simulink model "Flyback_converter"  (R2022b)
settings: Solver=ode23t  StartTime=0.0  StopTime=.2  RelTol=1e-3
libraries: spsSeriesRLCBranchLib x5, spsCurrentMeasurementLib x2, spsVoltageMeasurementLib x2, spsDCVoltageSourceLib x1, spsDiodeLib x1, spsLinearTransformerLib x1, dspstat3 x1, spsMosfetLib x1, simulink x1, spspowerguiLib x1
settings Model: Creator=es-ahmedabdellatif20  LastModifiedBy=es-ahmedabdellatif20

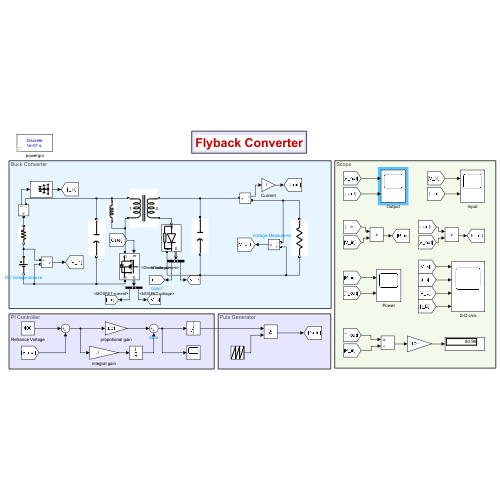
[thumbnail: Simulink's stored preview of the top-level diagram]
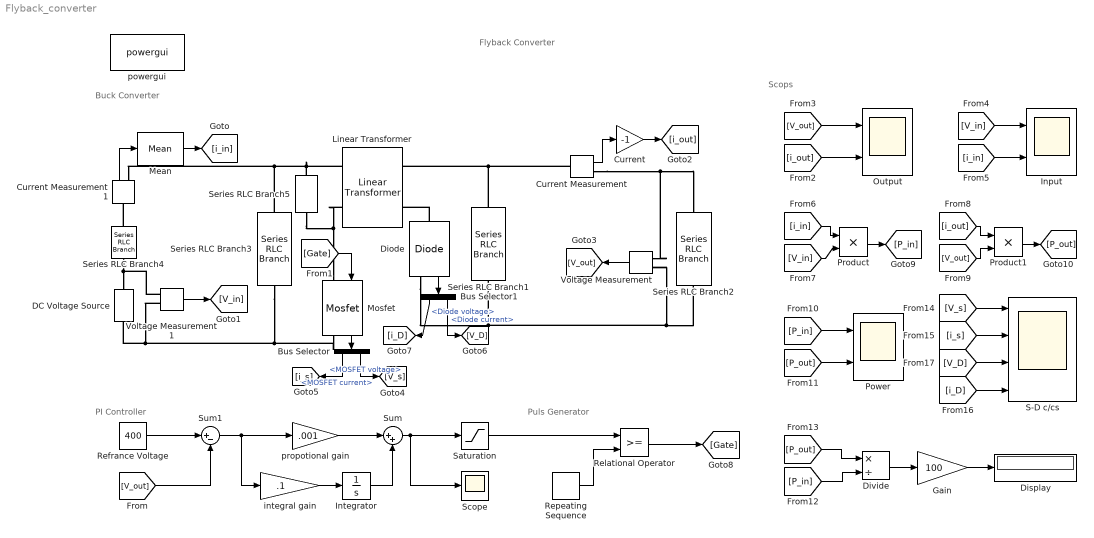
== system Flyback_converter ==
  note: Scops
  note: Flyback Converter
  note: Puls Generator
  note: PI Controller
  note: Buck Converter
  Bus Selector : BusSelector  OutputSignals=MOSFET current,MOSFET voltage
  Bus Selector1 : BusSelector  OutputSignals=Diode voltage,Diode current
  Current : Gain  Gain=-1
  Current Measurement : spsCurrentMeasurementLib/Current Measurement  PhasorSimulation=off  OutputType=Complex  PSBequivalent=0
  Current Measurement1 : spsCurrentMeasurementLib/Current Measurement  PhasorSimulation=off  OutputType=Complex  PSBequivalent=0
  DC Voltage Source : spsDCVoltageSourceLib/DC Voltage Source  Amplitude=800  Measurements=Voltage
  Diode : spsDiodeLib/Diode  Ron=0.001  Lon=0  Vf=0.8  IC=0  UseSnubber=0  Rs=500  Cs=250e-9  Measurements=on
  Display : Display
  Divide : Product  Inputs=*/
  Gain : Gain  Gain=100
  Input : Scope  NumInputPorts=2
  Integrator : Integrator
  Linear Transformer : spsLinearTransformerLib/Linear Transformer  UNITS=pu  NominalPower=[ 4000 250000 ]  winding1="[ 800  0  0 ]"  winding2="[ 400  0  0 ]"  ThreeWindings=off  winding3=[ 315e3 0.002 0.08 ]  RmLm=[ 500 0 ]  Measurements=None  DataType=off
  Mean : dspstat3/Mean  run=on  InputProcessing=Columns as channels (frame based)  reset_popup=None  directionMode=Each column  dimension=1  roiEnable=off  roiType=Rectangles  roiPortion=Entire ROI  roiOutput=Individual statistics for each ROI  roiFlag=off  roundingMode=Floor  overflowMode=off  outputDataTypeStr=Inherit: Same as accumulator  outputMin=[]  outputMax=[]  outputLastDataTypeStr=Inherit: Same as accumulator
  Mosfet : spsMosfetLib/Mosfet  Ron=0.1  Lon=0  Rd=0.01  Vfd=0  IC=0  Rs=1e5  Cs=inf  Measurements=on
  Output : Scope  NumInputPorts=2
  Power : Scope  NumInputPorts=2
  Product : Product
  Product1 : Product
  Refrance Voltage : Constant  Value=400
  Relational Operator : RelationalOperator  OutDataTypeStr=boolean  RndMeth=Simplest  InputSameDT=off
  Repeating Sequence : simulink/Sources/Repeating Sequence  rep_seq_t=[0 1/250000]  rep_seq_y=[0 1]
  S-D c/cs : Scope  NumInputPorts=4
  Saturation : Saturate  UpperLimit=1  LowerLimit=0
  Scope : Scope
  Series RLC Branch1 : spsSeriesRLCBranchLib/Series RLC Branch  LConnTagsString=__new0  RConnTagsString=__new0  BranchType=C  Resistance=1  Inductance=1e-3  SetiL0=off  InitialCurrent=0  Capacitance=660e-6  Setx0=on  InitialVoltage=200  Measurements=None
  Series RLC Branch2 : spsSeriesRLCBranchLib/Series RLC Branch  LConnTagsString=__new0  RConnTagsString=__new0  BranchType=R  Resistance=22.5  Inductance=1e-3  SetiL0=off  InitialCurrent=0  Capacitance=1e-6  Setx0=off  InitialVoltage=0  Measurements=None
  Series RLC Branch3 : spsSeriesRLCBranchLib/Series RLC Branch  LConnTagsString=__new0  RConnTagsString=__new0  BranchType=C  Resistance=1  Inductance=1e-3  SetiL0=off  InitialCurrent=0  Capacitance=1000e-6  Setx0=on  InitialVoltage=400  Measurements=None
  Series RLC Branch4 : spsSeriesRLCBranchLib/Series RLC Branch  LConnTagsString=__new0  RConnTagsString=__new0  BranchType=R  Resistance=.001  Inductance=1e-3  SetiL0=off  InitialCurrent=0  Capacitance=1000e-6  Setx0=off  InitialVoltage=0  Measurements=None
  Series RLC Branch5 : spsSeriesRLCBranchLib/Series RLC Branch  LConnTagsString=__new0  RConnTagsString=__new0  BranchType=L  Resistance=1  Inductance=100e-6  SetiL0=off  InitialCurrent=0  Capacitance=660e-6  Setx0=off  InitialVoltage=0  Measurements=None
  Sum : Sum  Inputs=|++
  Sum1 : Sum  Inputs=|+-
  Voltage Measurement : spsVoltageMeasurementLib/Voltage Measurement  PhasorSimulation=off  OutputType=Complex  PSBequivalent=0
  Voltage Measurement1 : spsVoltageMeasurementLib/Voltage Measurement  PhasorSimulation=off  OutputType=Complex  PSBequivalent=0
  integral gain : Gain  Gain=.1
  powergui : spspowerguiLib/powergui  Priority=1  SimulationMode=Discrete  SampleTime=1e-7  frequency=60  Iterations=50  frequencyindice=0  Pbase=100e6  ErrMax=1e-4  UnitsV=kV  UnitsW=MW  buscounter=0  FunctionMessages=off  echomessages=off  EnableUseOfTLC=off  CurrentSourceSwitches=off  DisableSnubberDevices=off  DisableRonSwitches=off  DisableVfSwitches=off  DisplayEquations=off  AutomaticDiscreteSolvers=off  SolverType=Tustin/Backward Euler (TBE)  Interpol=off  ExternalGateDelay=off  methode=off  Ts=100  x0status=blocks  SPID=on  SwTol=0  HookPort=off  NonlinearTolerance=1e-4  nMaxIteration=100  ContinueOnMaxIteration=off  RestoreLinks=warning  ResistiveCurrentMeasurement=off  Frange=[0:2:500]  Ylog=off  Xlog=on  ShowGrid=off  save=off  variable=ZData  structure=0  ZoomFFT=off  StartTime=0.0  cycles=1  DisplayStyle=1  fundamental=60  FreqAxis=off  MaxFrequency=1000  frequencyindicesteady=1  RmsSteady=1  display=off
  propotional gain : Gain  Gain=.001
  wires:
  Voltage Measurement1/1 -> [V_in]
  Voltage Measurement/1 -> [V_out]
  integral gain/1 -> Integrator/1
  Integrator/1 -> Sum/2
  propotional gain/1 -> Sum/1
  Sum/1 -> Scope/1, Saturation/1
  Relational Operator/1 -> [Gate]
  Refrance Voltage/1 -> Sum1/1
  [V_out] -> Sum1/2
  Sum1/1 -> integral gain/1, propotional gain/1
  Repeating Sequence/1 -> Relational Operator/2
  [V_out] -> Output/1
  [i_out] -> Output/2
  [i_in] -> Input/2
  [V_in] -> Input/1
  [i_in] -> Product/1
  [V_in] -> Product/2
  [V_out] -> Product1/2
  [i_out] -> Product1/1
  Product/1 -> [P_in]
  Product1/1 -> [P_out]
  [P_in] -> Power/1
  [P_out] -> Power/2
  [P_out] -> Divide/1
  [P_in] -> Divide/2
  Divide/1 -> Gain/1
  Gain/1 -> Display/1
  [V_s] -> S-D c/cs/1
  [i_s] -> S-D c/cs/2
  [V_D] -> S-D c/cs/3
  [i_D] -> S-D c/cs/4
  Current Measurement1/1 -> Mean/1
  Mean/1 -> [i_in]
  [Gate] -> Mosfet/1
  Mosfet/1 -> Bus Selector/1
  Bus Selector/1 -> [i_s]  "<MOSFET current>"
  Bus Selector/2 -> [V_s]  "<MOSFET voltage>"
  Saturation/1 -> Relational Operator/1
  Current Measurement/1 -> Current/1
  Current/1 -> [i_out]
  Diode/1 -> Bus Selector1/1
  Bus Selector1/2 -> [V_D]  "<Diode current>"
  Bus Selector1/1 -> [i_D]  "<Diode voltage>"
  connections:
  Voltage Measurement1/LConn2 -- DC Voltage Source/LConn1 -- Series RLC Branch3/RConn1 -- Mosfet/RConn1
  Voltage Measurement1/LConn1 -- Series RLC Branch4/RConn1 -- DC Voltage Source/RConn1
  Series RLC Branch3/LConn1 -- Series RLC Branch5/LConn1 -- Linear Transformer/LConn1 -- Current Measurement1/RConn1
  Linear Transformer/LConn2 -- Series RLC Branch5/RConn1 -- Mosfet/LConn1
  Diode/LConn1 -- Linear Transformer/RConn2
  Series RLC Branch1/LConn1 -- Linear Transformer/RConn1 -- Current Measurement/LConn1
  Diode/RConn1 -- Voltage Measurement/LConn1 -- Series RLC Branch2/RConn1 -- Series RLC Branch1/RConn1
  Current Measurement/RConn1 -- Series RLC Branch2/LConn1 -- Voltage Measurement/LConn2
  Series RLC Branch4/LConn1 -- Current Measurement1/LConn1
